simulink model "digitalDesign_ester"  (R2025b)
settings: Solver=FixedStepAuto  StartTime=0.0  StopTime=10  FixedStep=0.0001  RelTol=1e-3
values from neighbouring files (symbols this model uses):
  Beq = B_eq_est    [lab2_directDigitalDesign_ester.m]    (also in lab2_pidDT_ester.m; lab2_ssCT_ester.m; lab2_ssDT_ester.m)
  gamma_o = [gamma(2)-L*gamma(1), (phi22-L*phi12)*L+phi21-L*phi11]    [lab2_directDigitalDesign_ester.m]    (also in lab2_ssDT_ester.m = phi_o*Bo*T)
  Ho = [0;1]    [lab2_directDigitalDesign_ester.m]    (also in lab2_ssDT_ester.m = Co*phi_o)
  Jeq = J_eq_est    [lab2_directDigitalDesign_ester.m]    (also in lab2_pidDT_ester.m; lab2_ssCT_ester.m; lab2_ssDT_ester.m)
  Jo = [0 1; 0 L]    [lab2_directDigitalDesign_ester.m]    (also in lab2_ssDT_ester.m = Do+Co*phi_o*Bo*T)
  K = Ke(2:3)    [lab2_directDigitalDesign_ester.m]    (also in lab2_ssCT_ester.m = K2; lab2_ssDT_ester.m = K2)
  Ki = Ke(1)    [lab2_directDigitalDesign_ester.m]    (also in lab2_ssCT_ester.m = 0; lab2_ssDT_ester.m = 0)
  Nr = Nu + K * Nx    [lab2_directDigitalDesign_ester.m]    (also in lab2_ssCT_ester.m = Nr2; lab2_ssDT_ester.m = Nr2)
  phi_o = lambda_o_dt    [lab2_directDigitalDesign_ester.m]    (also in lab2_ssDT_ester.m = 1/(1-Ao*T))
  step_amplitude = 50    [lab2_directDigitalDesign_ester.m]    (also in lab2_pidDT_ester.m = 360; lab2_ssDT_ester.m)
  T = input('Select sample time (0.001, 0.01, 0.05) [s]: ')    [lab2_directDigitalDesign_ester.m]    (also in lab2_pidDT_ester.m; lab2_ssCT_ester.m = sampleTime_options(1); lab2_ssDT_ester.m)
undefined symbols (not defined in the file or in its folder): DiscIntNeverNeededParam, drv, gbox, mld, mot, rads2rpm, Req
settings Model: Creator=ester  LastModifiedBy=ester

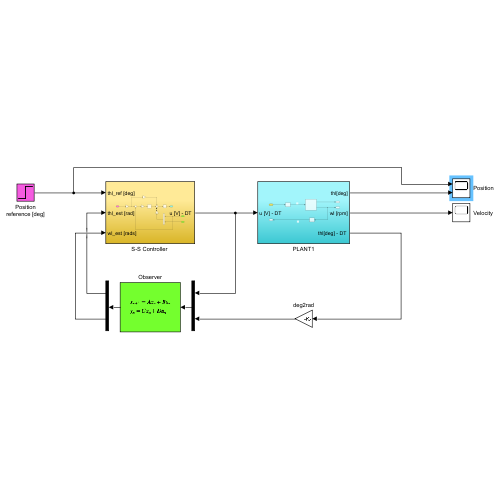
[thumbnail: Simulink's stored preview of the top-level diagram]
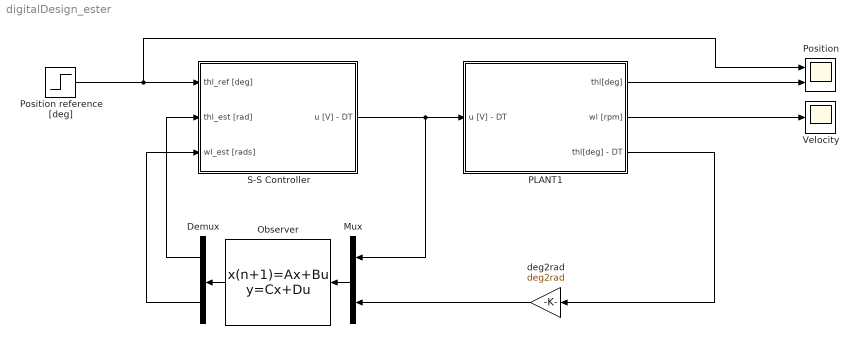
== system digitalDesign_ester ==
  Demux : Demux  Outputs=2
  Mux : Mux  Inputs=2
  Observer : DiscreteStateSpace  A=phi_o  B=gamma_o  C=Ho  D=Jo  SampleTime=T
  PLANT1 : Subsystem
  Position : Scope  NumInputPorts=2
      settings: ActiveDisplayYMinimum=-9.4053833831629419  ActiveDisplayYMaximum=84.648450448466491
  Position reference [deg] : Step  After=step_amplitude  SampleTime=T  ZeroCross=off
  "S-S Controller " : Subsystem
  Velocity : Scope
      settings: ActiveDisplayYMinimum=-1  ActiveDisplayYMaximum=1
  deg2rad : Gain  Gain=deg2rad
  wires:
  Position reference [deg]/1 -> "S-S Controller "/1(thl_ref [deg]), Position/1
  deg2rad/1 -> Mux/2
  PLANT1/3("thl[deg] - DT ") -> deg2rad/1
  "S-S Controller "/1("u [V] - DT ") -> PLANT1/1(u [V] - DT), Mux/1
  Observer/1 -> Demux/1
  Demux/2 -> "S-S Controller "/3(wl_est [rads])
  Demux/1 -> "S-S Controller "/2(thl_est [rad])
  PLANT1/1(thl[deg]) -> Position/2
  Mux/1 -> Observer/1
  PLANT1/2(wl [rpm]) -> Velocity/1

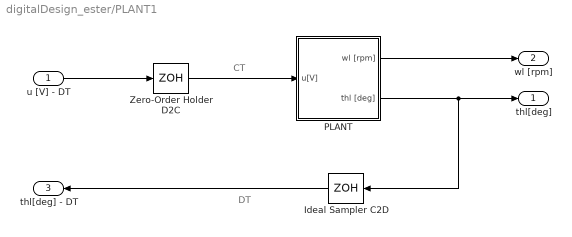
== system digitalDesign_ester/PLANT1 ==
  note: DT
  note: CT
  u [V] - DT : Inport
  Ideal Sampler C2D : ZeroOrderHold  SampleTime=T
  PLANT : Subsystem
  Zero-Order Holder D2C : ZeroOrderHold  SampleTime=T
  thl[deg] : Outport
  wl [rpm] : Outport  Port=2
  "thl[deg] - DT " : Outport  Port=3
  wires:
  PLANT/2(thl [deg]) -> Ideal Sampler C2D/1, thl[deg]/1
  Ideal Sampler C2D/1 -> "thl[deg] - DT "/1
  u [V] - DT/1 -> Zero-Order Holder D2C/1
  PLANT/1(wl [rpm]) -> wl [rpm]/1
  Zero-Order Holder D2C/1 -> PLANT/1(u[V])

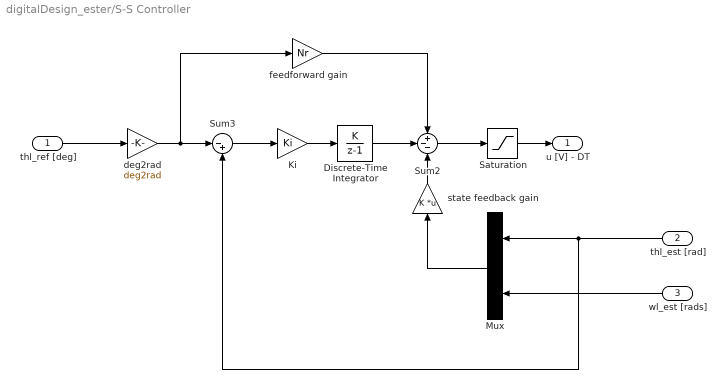
== system digitalDesign_ester/S-S Controller  ==
  thl_ref [deg] : Inport
  thl_est [rad] : Inport  Port=2
  wl_est [rads] : Inport  Port=3
  " feedforward gain" : Gain  Gain=Nr
  Discrete-Time Integrator : DiscreteIntegrator  IntegratorMethod=Accumulation: Forward Euler  SampleTime=T  ICPrevOutput=DiscIntNeverNeededParam  ICPrevScaledInput=DiscIntNeverNeededParam
  Ki : Gain  Gain=Ki
  Mux : Mux  Inputs=2
  Saturation : Saturate  UpperLimit=10  LowerLimit=-10  ZeroCross=off
  Sum2 : Sum  Inputs=+--
  Sum3 : Sum  Inputs=|-+
  deg2rad : Gain  Gain=deg2rad
  state feedback gain : Gain  Gain=K  Multiplication=Matrix(K*u)
  "u [V] - DT " : Outport
  wires:
  Mux/1 -> state feedback gain/1
  Ki/1 -> Discrete-Time Integrator/1
  deg2rad/1 -> " feedforward gain"/1, Sum3/1
  Sum2/1 -> Saturation/1
  Saturation/1 -> "u [V] - DT "/1
  thl_est [rad]/1 -> Sum3/2, Mux/1
  Sum3/1 -> Ki/1
  state feedback gain/1 -> Sum2/3
  " feedforward gain"/1 -> Sum2/1
  thl_ref [deg]/1 -> deg2rad/1
  wl_est [rads]/1 -> Mux/2
  Discrete-Time Integrator/1 -> Sum2/2

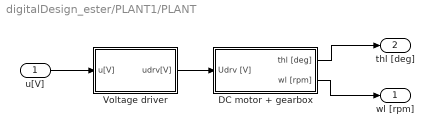
== system digitalDesign_ester/PLANT1/PLANT ==
  u[V] : Inport
  DC motor + gearbox : Subsystem
  Voltage driver : Subsystem  TreatAsAtomicUnit=on
  wl [rpm] : Outport
  thl [deg] : Outport  Port=2
  wires:
  Voltage driver/1(udrv[V]) -> DC motor + gearbox/1(Udrv [V])
  u[V]/1 -> Voltage driver/1(u[V])
  DC motor + gearbox/1(thl [deg]) -> thl [deg]/1
  DC motor + gearbox/2(wl [rpm]) -> wl [rpm]/1

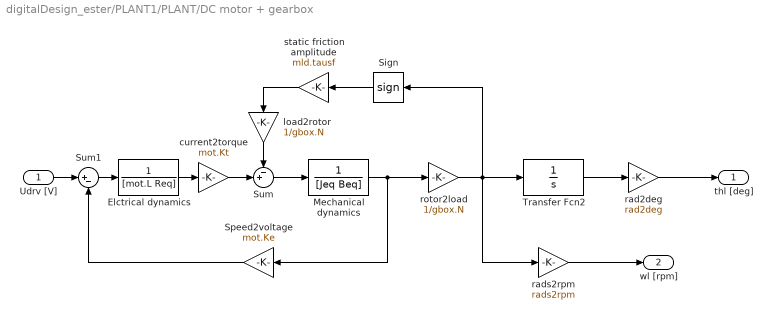
== system digitalDesign_ester/PLANT1/PLANT/DC motor + gearbox ==
  Udrv [V] : Inport
  Elctrical dynamics : TransferFcn  Denominator=[mot.L Req]
  Mechanical dynamics : TransferFcn  Denominator=[Jeq Beq]
  Sign : Signum  ZeroCross=off
  Speed2voltage : Gain  Gain=mot.Ke
  Sum : Sum  Inputs=-+|
  Sum1 : Sum  Inputs=|+-
  Transfer Fcn2 : TransferFcn  Denominator=[1 0]
  current2torque : Gain  Gain=mot.Kt
  load2rotor : Gain  Gain=1/gbox.N
  rad2deg : Gain  Gain=rad2deg
  rads2rpm : Gain  Gain=rads2rpm
  rotor2load : Gain  Gain=1/gbox.N
  static friction amplitude : Gain  Gain=mld.tausf
  thl [deg] : Outport
  wl [rpm] : Outport  Port=2
  wires:
  rotor2load/1 -> Sign/1, rads2rpm/1, Transfer Fcn2/1
  Sign/1 -> static friction amplitude/1
  rads2rpm/1 -> wl [rpm]/1
  Sum/1 -> Mechanical dynamics/1
  Udrv [V]/1 -> Sum1/1
  static friction amplitude/1 -> load2rotor/1
  load2rotor/1 -> Sum/1
  Transfer Fcn2/1 -> rad2deg/1
  current2torque/1 -> Sum/2
  Speed2voltage/1 -> Sum1/2
  Mechanical dynamics/1 -> Speed2voltage/1, rotor2load/1
  Elctrical dynamics/1 -> current2torque/1
  Sum1/1 -> Elctrical dynamics/1
  rad2deg/1 -> thl [deg]/1

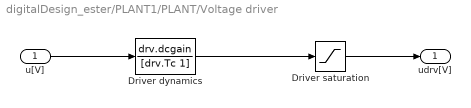
== system digitalDesign_ester/PLANT1/PLANT/Voltage driver ==
  u[V] : Inport
  Driver dynamics : TransferFcn  Numerator=drv.dcgain  Denominator=[drv.Tc 1]
  Driver saturation : Saturate  UpperLimit=drv.outmax  LowerLimit=-drv.outmax
  udrv[V] : Outport
  wires:
  Driver dynamics/1 -> Driver saturation/1
  u[V]/1 -> Driver dynamics/1
  Driver saturation/1 -> udrv[V]/1
